simulink model "gpc_siso_1_sim"  (R2022a)
settings: Solver=VariableStepAuto  StartTime=0.0  StopTime=20  RelTol=1e-3
undefined symbols (not defined in the file): a, A, b, B, D, delta, F, H, K, Kr, Ts
settings Model: Creator=aaron  LastModifiedBy=aaron
settings SolverCC: AlgebraicLoopSolver=TrustRegion
settings DebuggingCC: UnconnectedInputMsg=warning  UnconnectedOutputMsg=warning  UnconnectedLineMsg=warning  SFMachineParentedDataDiag=warning

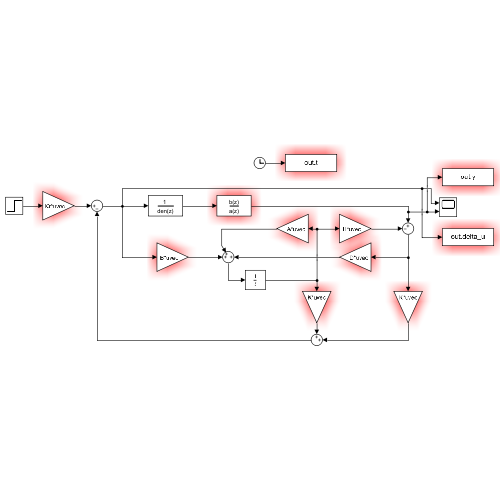
[thumbnail: Simulink's stored preview of the top-level diagram]
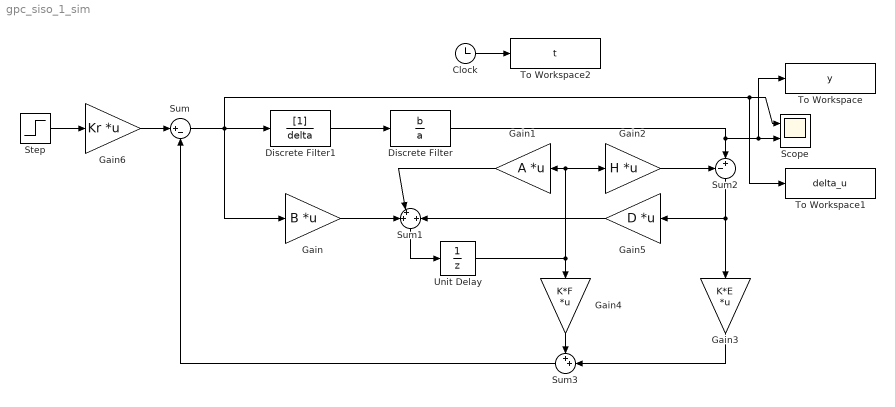
== system gpc_siso_1_sim ==
  Clock : Clock
  Discrete Filter : DiscreteFilter  Numerator=b  Denominator=a
  Discrete Filter1 : DiscreteFilter  Denominator=delta
  Gain : Gain  Gain=B  Multiplication=Matrix(K*u) (u vector)
  Gain1 : Gain  Gain=A  Multiplication=Matrix(K*u) (u vector)
  Gain2 : Gain  Gain=H  Multiplication=Matrix(K*u) (u vector)
  Gain3 : Gain  Gain=K*E  Multiplication=Matrix(K*u) (u vector)
  Gain4 : Gain  Gain=K*F  Multiplication=Matrix(K*u) (u vector)
  Gain5 : Gain  Gain=D  Multiplication=Matrix(K*u) (u vector)
  Gain6 : Gain  Gain=Kr  Multiplication=Matrix(K*u) (u vector)
  Scope : Scope  NumInputPorts=2
  Step : Step  Time=0  SampleTime=0
  Sum : Sum  Inputs=|+-
  Sum1 : Sum  Inputs=++|+
  Sum2 : Sum  Inputs=-+|
  Sum3 : Sum  Inputs=++|
  To Workspace : ToWorkspace  VariableName=y  SampleTime=Ts
  To Workspace1 : ToWorkspace  VariableName=delta_u  SampleTime=Ts
  To Workspace2 : ToWorkspace  VariableName=t  SampleTime=Ts
  Unit Delay : UnitDelay  SampleTime=-1  HasFrameUpgradeWarning=on
  wires:
  Discrete Filter1/1 -> Discrete Filter/1
  Step/1 -> Gain6/1
  Gain/1 -> Sum1/1
  Sum1/1 -> Unit Delay/1
  Gain1/1 -> Sum1/2
  Unit Delay/1 -> Gain4/1, Gain2/1, Gain1/1
  Gain2/1 -> Sum2/1
  Sum2/1 -> Gain5/1, Gain3/1
  Gain5/1 -> Sum1/3
  Gain4/1 -> Sum3/1
  Gain3/1 -> Sum3/2
  Sum3/1 -> Sum/2
  Gain6/1 -> Sum/1
  Discrete Filter/1 -> Sum2/2, Scope/2, To Workspace/1
  Clock/1 -> To Workspace2/1
  Sum/1 -> Gain/1, To Workspace1/1, Scope/1, Discrete Filter1/1
